simulink model "Current_Control"  (R2013a)
settings: Solver=ode45  StartTime=0.0  StopTime=0.02  MaxStep=1e-4  RelTol=1e-3
values from neighbouring files (symbols this model uses):
  kf = 0.35    [Plot3.m]    (also in Plot4.m; Q10.m; Q6.m; Q9.m)
  kic = alphac^2*La    (= 24674.0110027)    [Plot3.m]    (also in Plot4.m; Q10.m; Q6.m; Q9.m = 17271.8077019)
  kpc = alphac*La    (= 7.85398163397)    [Plot3.m]    (also in Plot4.m; Q10.m; Q6.m; Q9.m = 5.49778714378)
  r = kpc - Ra    (= 7.35398163397)    [Plot3.m]    (also in Plot4.m; Q10.m; Q6.m; Q9.m = 4.74778714378)
  Umax = 140    [Plot3.m]    (also in Plot4.m; Q10.m; Q6.m; Q9.m)
  Umin = -140    [Plot3.m]    (also in Plot4.m; Q10.m; Q6.m; Q9.m)
settings Model: Creator=Sony  LastModifiedBy=Sony

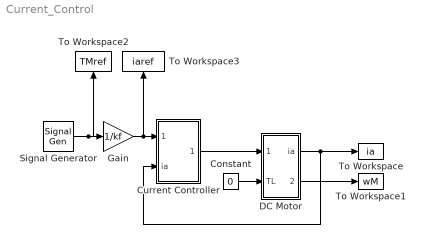
== system Current_Control ==
  Constant : Constant  Value=0
  Current Controller : Subsystem
  DC Motor : Subsystem  mask{Ra=0.5, La=2.5e-3, kf=0.35, J=1e-3}
      mask prompts: Ra "Ra (ohm)"; La "La (H)"; kf "kf (Vs)"; J "J (kgm^2)"
  Gain : Gain  Gain=1/kf
  Signal Generator : SignalGenerator  WaveForm=square  Frequency=100
  To Workspace : ToWorkspace  VariableName=ia  SampleTime=-1  SaveFormat=Timeseries
  To Workspace1 : ToWorkspace  VariableName=wM  SampleTime=-1  SaveFormat=Timeseries
  To Workspace2 : ToWorkspace  VariableName=TMref  SampleTime=-1  SaveFormat=Timeseries
  To Workspace3 : ToWorkspace  VariableName=iaref  SampleTime=-1  SaveFormat=Timeseries
  wires:
  DC Motor/1(ia) -> Current Controller/2(ia), To Workspace/1
  DC Motor/2(wM) -> To Workspace1/1
  Constant/1 -> DC Motor/2(TL)
  Signal Generator/1 -> To Workspace2/1, Gain/1
  Current Controller/1(uaref) -> DC Motor/1(ua)
  Gain/1 -> To Workspace3/1, Current Controller/1(iaref)

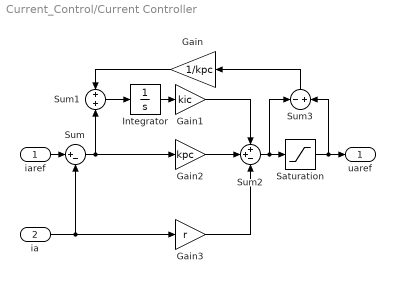
== system Current_Control/Current Controller ==
  iaref : Inport
  ia : Inport  Port=2
  Gain : Gain  Gain=1/kpc
  Gain1 : Gain  Gain=kic
  Gain2 : Gain  Gain=kpc
  Gain3 : Gain  Gain=r
  Integrator : Integrator
  Saturation : Saturate  UpperLimit=Umax  LowerLimit=Umin
  Sum : Sum  Inputs=|+-
  Sum1 : Sum  Inputs=+|+
  Sum2 : Sum  Inputs=++-
  Sum3 : Sum  Inputs=-|+
  uaref : Outport
  wires:
  Sum1/1 -> Integrator/1
  Gain/1 -> Sum1/1
  Integrator/1 -> Gain1/1
  iaref/1 -> Sum/1
  Sum/1 -> Gain2/1, Sum1/2
  Gain2/1 -> Sum2/2
  Gain1/1 -> Sum2/1
  ia/1 -> Gain3/1, Sum/2
  Gain3/1 -> Sum2/3
  Sum3/1 -> Gain/1
  Sum2/1 -> Sum3/1, Saturation/1
  Saturation/1 -> Sum3/2, uaref/1

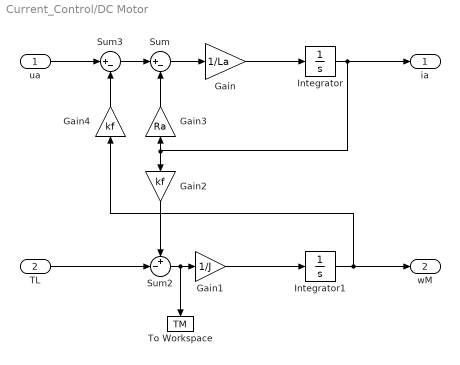
== system Current_Control/DC Motor ==
  ua : Inport
  TL : Inport  Port=2
  Gain : Gain  Gain=1/La
  Gain1 : Gain  Gain=1/J
  Gain2 : Gain  Gain=kf
  Gain3 : Gain  Gain=Ra
  Gain4 : Gain  Gain=kf
  Integrator : Integrator
  Integrator1 : Integrator
  Sum : Sum  Inputs=|+-
  Sum2 : Sum  Inputs=+-|
  Sum3 : Sum  Inputs=|+-
  To Workspace : ToWorkspace  VariableName=TM  SampleTime=-1  SaveFormat=Timeseries
  ia : Outport
  wM : Outport  Port=2
  wires:
  Gain3/1 -> Sum/2
  Gain1/1 -> Integrator1/1
  Integrator/1 -> ia/1, Gain2/1, Gain3/1
  Sum2/1 -> To Workspace/1, Gain1/1
  Sum3/1 -> Sum/1
  Sum/1 -> Gain/1
  TL/1 -> Sum2/2
  Gain4/1 -> Sum3/2
  Integrator1/1 -> wM/1, Gain4/1
  Gain2/1 -> Sum2/1
  ua/1 -> Sum3/1
  Gain/1 -> Integrator/1
